simulink model "prob6"  (R2020b)
settings: Solver=VariableStepAuto  StartTime=0.0  StopTime=10.0  RelTol=1e-3
settings Model: Creator=Nitin  LastModifiedBy=Nitin

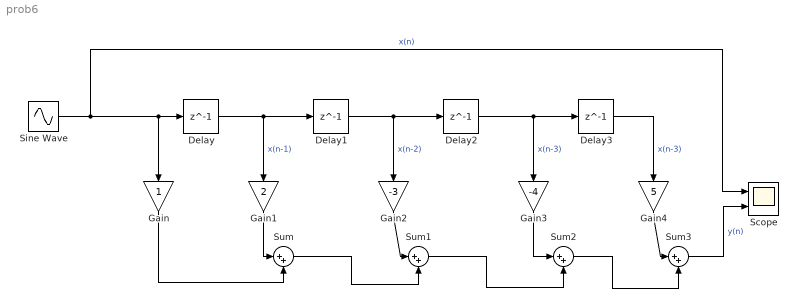
== system prob6 ==
  Delay{,1..3} (4 alike) : Delay  DelayLength=1
  Gain : Gain
  Gain1 : Gain  Gain=2
  Gain2 : Gain  Gain=-3
  Gain3 : Gain  Gain=-4
  Gain4 : Gain  Gain=5
  Scope : Scope  NumInputPorts=2
  Sine Wave : Sin  SampleTime=0
  Sum{,1..3} (4 alike) : Sum  Inputs=|++
  wires:
  Delay/1 -> Gain1/1, Delay1/1  "x(n-1)"
  Sum2/1 -> Sum3/2
  Sum3/1 -> Scope/2  "y(n)"
  Delay3/1 -> Gain4/1  "x(n-3)"
  Sine Wave/1 -> Scope/1, Gain/1, Delay/1  "x(n)"
  Sum/1 -> Sum1/2
  Gain/1 -> Sum/2
  Gain1/1 -> Sum/1
  Sum1/1 -> Sum2/2
  Gain2/1 -> Sum1/1
  Delay1/1 -> Gain2/1, Delay2/1  "x(n-2)"
  Gain4/1 -> Sum3/1
  Gain3/1 -> Sum2/1
  Delay2/1 -> Gain3/1, Delay3/1  "x(n-3)"
